simulink model "planar_quad_animation"  (R2017a)
settings: Solver=ode45  StartTime=0.0  StopTime=inf  RelTol=1e-3  EnableMultiTasking=on
undefined symbols (not defined in the file or in its folder): drawPlanarQuad
libraries: simulink x4
settings Model: Creator=ecestudent  LastModifiedBy=jesse
settings DataIOCC: LimitDataPoints=on  SaveFormat=Array
settings OptimizationCC: LifeSpan=inf
settings DebuggingCC: SFUnexpectedBacktrackingDiag=warning  SFNoUnconditionalDefaultTransitionDiag=warning  SFExecutionAtInitializationDiag=none
settings HardwareCC: ProdBitPerPointer=32  ProdBitPerSizeT=32  ProdBitPerPtrDiffT=32  ProdLargestAtomicFloat=None  ProdIntDivRoundTo=Undefined  ProdEndianess=Unspecified  ProdWordSize=32  ProdHWDeviceType=32-bit Generic
settings ModelReferenceCC: PropagateSignalLabelsOutOfModel=off
settings GRTTargetCC: TargetLangStandard=C89/C90 (ANSI)  GeneratePreprocessorConditionals=Disable all
settings ConfigComp: CovMetricSettings=dw  CovHtmlReporting=on  CovSaveCumulativeToWorkspaceVar=on  CovSaveSingleToWorkspaceVar=on  CovExternalEMLEnable=off

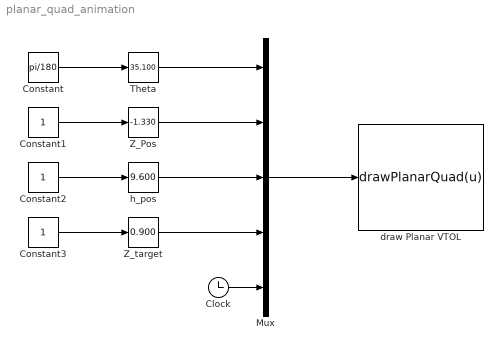
== system planar_quad_animation ==
  Clock : Clock
  Constant : Constant  Value=pi/180
  Constant1 : Constant
  Constant2 : Constant
  Constant3 : Constant
  Mux : Mux  Inputs=5
  Theta : simulink/Math Operations/Slider Gain  gain=35.100  low=-45  high=45
  Z_Pos : simulink/Math Operations/Slider Gain  gain=-1.330  low=-3.5  high=3.5
  Z_target : simulink/Math Operations/Slider Gain  gain=0.900  low=-5  high=5
  draw Planar VTOL : MATLABFcn  MATLABFcn=drawPlanarQuad(u)  OutputDimensions=0
      mask Display: image(imread('tv.jpg'))
  h_pos : simulink/Math Operations/Slider Gain  gain=9.600  low=0  high=10
  wires:
  Constant/1 -> Theta/1
  Constant1/1 -> Z_Pos/1
  Constant2/1 -> h_pos/1
  Theta/1 -> Mux/1
  Z_Pos/1 -> Mux/2
  h_pos/1 -> Mux/3
  Clock/1 -> Mux/5
  Mux/1 -> draw Planar VTOL/1
  Z_target/1 -> Mux/4
  Constant3/1 -> Z_target/1
